simulink model "DIME12_Ctrl_dSpaceHRBMAB"  (R2018b)
settings: Solver=ode1  StartTime=0.0  StopTime=inf  FixedStep=0.5  RelTol=1e-3
PostLoadFcn:
  | if any(exist('dsrtsu_mdlpostloadfcn', 'file') ~= 0), dsrtsu_mdlpostloadfcn('Execute', bdroot); end
InitFcn:
  | , if any(exist('dsmpb_private', 'file') ~= 0), dsmpb_private('dsmpb_mdlclblib', 'Init', bdroot); end,
  | load('LUT_PSM.mat')
  | load('Torque_ts.mat')
  | 
  | p = 1;
  | L_q = 1.575e-3;
  | L_d = L_q;
  | Psi_M = 0.0353*2*pi;
  | R_s = 639e-3;
  | Ts = 1/40e3;
  | J_ges = 9.56e-5;
  | d_viskos = 0.01;
  | mpsTestMaxVelocityDmd = 166.7;
  | mpsTestVelocityDmd = 0;
  | EDC_CURRENT_CONTROL_EXECUTION_PERIOD = 4e-5;
  | 
undefined symbols (not defined in the file or in its folder): d, motor_KF, Psidq, Psiqd, q, SimSampleT
libraries: simulink x37, dsmpblib x12, simulink_extras x3
(part 2 of 2)

== system DIME12_Ctrl_dSpaceHRBMAB/DIME Regler/Controller/speed_controller/DISCRETE_PT1_SET ==
  Reset[0|1] : Inport
  In : Inport  Port=2
  K : Inport  Port=3
  T[s] : Inport  Port=4
  T_Sample[s] : Inport  Port=5
  1|FilterTime : Product  Inputs=*/  SaturateOnIntegerOverflow=on  InputSameDT=on  OutDataTypeStr=Inherit: Same as first input
  Proportional : Product  Inputs=**  SaturateOnIntegerOverflow=on  InputSameDT=on  OutDataTypeStr=Inherit: Same as first input
  Sum : Sum  Inputs=-+|  SaturateOnIntegerOverflow=on  InputSameDT=on  OutDataTypeStr=Inherit: Same as first input
  Unit Delay : UnitDelay  SampleTime=-1
  discrete_Integrator_Init : Subsystem
  zero : Constant  Value=0  SampleTime=-1
  Out : Outport
  wires:
  zero/1 -> discrete_Integrator_Init/3(Initial)
  T_Sample[s]/1 -> discrete_Integrator_Init/4(T_Sample[s])
  Reset[0|1]/1 -> discrete_Integrator_Init/1(Reset[0|1])
  T[s]/1 -> 1|FilterTime/2
  Unit Delay/1 -> Sum/1
  1|FilterTime/1 -> Unit Delay/1, Out/1
  discrete_Integrator_Init/1(Out) -> 1|FilterTime/1
  Proportional/1 -> Sum/2
  K/1 -> Proportional/2
  Sum/1 -> discrete_Integrator_Init/2(In)
  In/1 -> Proportional/1

== system DIME12_Ctrl_dSpaceHRBMAB/DIME Regler/Controller/speed_controller/DISCRETE_PT1_SET1 ==
  Reset[0|1] : Inport
  In : Inport  Port=2
  K : Inport  Port=3
  T[s] : Inport  Port=4
  T_Sample[s] : Inport  Port=5
  1|FilterTime : Product  Inputs=*/  SaturateOnIntegerOverflow=on  InputSameDT=on  OutDataTypeStr=Inherit: Same as first input
  Proportional : Product  Inputs=**  SaturateOnIntegerOverflow=on  InputSameDT=on  OutDataTypeStr=Inherit: Same as first input
  Sum : Sum  Inputs=-+|  SaturateOnIntegerOverflow=on  InputSameDT=on  OutDataTypeStr=Inherit: Same as first input
  Unit Delay : UnitDelay  SampleTime=-1
  discrete_Integrator_Init : Subsystem
  zero : Constant  Value=0  SampleTime=-1
  Out : Outport
  wires:
  zero/1 -> discrete_Integrator_Init/3(Initial)
  T_Sample[s]/1 -> discrete_Integrator_Init/4(T_Sample[s])
  Reset[0|1]/1 -> discrete_Integrator_Init/1(Reset[0|1])
  T[s]/1 -> 1|FilterTime/2
  Unit Delay/1 -> Sum/1
  1|FilterTime/1 -> Unit Delay/1, Out/1
  discrete_Integrator_Init/1(Out) -> 1|FilterTime/1
  Proportional/1 -> Sum/2
  K/1 -> Proportional/2
  Sum/1 -> discrete_Integrator_Init/2(In)
  In/1 -> Proportional/1

== system DIME12_Ctrl_dSpaceHRBMAB/DIME Regler/Controller/speed_controller/Limit_n_Set ==
  In1 : Inport
  In2 : Inport  Port=2
  Saturation Dynamic : simulink/Discontinuities/Saturation Dynamic  OutMin=[]  OutMax=[]  OutDataTypeStr=Inherit: Same as second input  OutDataType=sfix(16)  OutScaling=2^-10  DoSatur=off
  inv : Gain  Gain=-1
  Out1 : Outport
  wires:
  inv/1 -> Saturation Dynamic/3
  In2/1 -> Saturation Dynamic/1, inv/1
  In1/1 -> Saturation Dynamic/2
  Saturation Dynamic/1 -> Out1/1

== system DIME12_Ctrl_dSpaceHRBMAB/DIME Regler/Controller/speed_controller/PI_CONTROLLER ==
  ActualValue : Inport
  RefValue : Inport  Port=2
  Kp : Inport  Port=3
  Ki : Inport  Port=4
  Limit_up : Inport  Port=5
  Limit_lo : Inport  Port=6
  T_Sample[s] : Inport  Port=7
  Product : Product  RndMeth=Zero
  Product1 : Product  RndMeth=Zero
  Product2 : Product  RndMeth=Zero
  Saturation Dynamic : simulink/Discontinuities/Saturation Dynamic  OutMin=[]  OutMax=[]  OutDataTypeStr=Inherit: Same as second input  OutDataType=sfix(16)  OutScaling=2^-10  DoSatur=off
  Sum : Sum  Inputs=+++  SaturateOnIntegerOverflow=on
  Sum1 : Sum  Inputs=+-  SaturateOnIntegerOverflow=on
  Sum2 : Sum  Inputs=-+|  SaturateOnIntegerOverflow=on
  Unit Delay : UnitDelay  SampleTime=-1
  y : Outport
  wires:
  Limit_lo/1 -> Saturation Dynamic/3
  Limit_up/1 -> Saturation Dynamic/1
  Sum/1 -> Saturation Dynamic/2
  Sum1/1 -> Product1/2, Product2/1  "error"
  RefValue/1 -> Sum1/1
  ActualValue/1 -> Sum1/2
  Product1/1 -> Sum/1, Sum2/1
  Product/1 -> Sum/2  "integral"
  Saturation Dynamic/1 -> Sum2/2, y/1
  Product2/1 -> Product/1
  Unit Delay/1 -> Sum/3
  Sum2/1 -> Unit Delay/1
  T_Sample[s]/1 -> Product/2
  Kp/1 -> Product1/1
  Ki/1 -> Product2/2

== system DIME12_Ctrl_dSpaceHRBMAB/DIME Regler/Controller/speed_controller/SignalCollector ==
  n_Limit[rpm] : Inport
  n[rpm] : Inport  Port=2
  n_Set[rpm] : Inport  Port=3
  Bus Creator : BusCreator  Inputs=3
  SignalBus : Outport
  wires:
  n_Limit[rpm]/1 -> Bus Creator/3  "n_Limit[rpm]"
  Bus Creator/1 -> SignalBus/1  "SPEED_CONTROLLER"
  n_Set[rpm]/1 -> Bus Creator/2  "n_Set[rpm]"
  n[rpm]/1 -> Bus Creator/1  "n[rpm]"

== system DIME12_Ctrl_dSpaceHRBMAB/DIME Regler/Outputs/Error Protection/current U ==
  Iphase1 : Inport
  CurrentNegLimit : Constant  Value=-18
  CurrentPosLimit : Constant  Value=18
  Logical Operator1 : Logic  Operator=OR  AllPortsSameDT=off  OutDataTypeStr=boolean
  current max : RelationalOperator  Operator=>  OutDataTypeStr=boolean  RndMeth=Simplest
  current min : RelationalOperator  Operator=<  OutDataTypeStr=boolean  RndMeth=Simplest
  Inverter_Current_U_Fault : Outport
  wires:
  Logical Operator1/1 -> Inverter_Current_U_Fault/1  "Inverter_Current_U_Fault"
  current min/1 -> Logical Operator1/2
  CurrentPosLimit/1 -> current max/2
  CurrentNegLimit/1 -> current min/2
  current max/1 -> Logical Operator1/1
  Iphase1/1 -> current min/1, current max/1

== system DIME12_Ctrl_dSpaceHRBMAB/DIME Regler/Outputs/Error Protection/current V ==
  Iphase2 : Inport
  CurrentNegLimit : Constant  Value=-18
  CurrentPosLimit : Constant  Value=18
  Logical Operator1 : Logic  Operator=OR  AllPortsSameDT=off  OutDataTypeStr=boolean
  current max : RelationalOperator  Operator=>  OutDataTypeStr=boolean  RndMeth=Simplest
  current min : RelationalOperator  Operator=<  OutDataTypeStr=boolean  RndMeth=Simplest
  Inverter_Current_V_Fault : Outport
  wires:
  Logical Operator1/1 -> Inverter_Current_V_Fault/1  "Inverter_Current_V_Fault"
  current min/1 -> Logical Operator1/2
  CurrentPosLimit/1 -> current max/2
  CurrentNegLimit/1 -> current min/2
  current max/1 -> Logical Operator1/1
  Iphase2/1 -> current min/1, current max/1

== system DIME12_Ctrl_dSpaceHRBMAB/DIME Regler/Outputs/Error Protection/current W ==
  Iphase3 : Inport
  CurrentNegLimit : Constant  Value=-18
  CurrentPosLimit : Constant  Value=18
  Logical Operator1 : Logic  Operator=OR  AllPortsSameDT=off  OutDataTypeStr=boolean
  current max : RelationalOperator  Operator=>  OutDataTypeStr=boolean  RndMeth=Simplest
  current min : RelationalOperator  Operator=<  OutDataTypeStr=boolean  RndMeth=Simplest
  Inverter_Current_W_Fault : Outport
  wires:
  Iphase3/1 -> current max/1, current min/1
  current max/1 -> Logical Operator1/1
  CurrentNegLimit/1 -> current min/2
  CurrentPosLimit/1 -> current max/2
  current min/1 -> Logical Operator1/2
  Logical Operator1/1 -> Inverter_Current_W_Fault/1  "Inverter_Current_W_Fault"

== system DIME12_Ctrl_dSpaceHRBMAB/DIME Regler/Outputs/Error Protection/speed ==
  meclVelocityMAB : Inport
  Logical Operator : Logic  Operator=OR  AllPortsSameDT=off  OutDataTypeStr=boolean
  SpeedNegLimit : Constant  Value=-10000/60
  SpeedPosLimit : Constant  Value=10000/60  OutDataTypeStr=double
  rpm max : RelationalOperator  Operator=>  OutDataTypeStr=boolean  RndMeth=Simplest
  rpm min : RelationalOperator  Operator=<  OutDataTypeStr=boolean  RndMeth=Simplest
  Engine_Speed_Fault : Outport
  wires:
  SpeedNegLimit/1 -> rpm min/2
  SpeedPosLimit/1 -> rpm max/2
  meclVelocityMAB/1 -> rpm min/1, rpm max/1
  rpm max/1 -> Logical Operator/1
  rpm min/1 -> Logical Operator/2
  Logical Operator/1 -> Engine_Speed_Fault/1  "Engine_Speed_Fault"

== system DIME12_Ctrl_dSpaceHRBMAB/DIME Regler/Outputs/Error Protection/termperature ==
  Temperature : Inport
  Relational Operator : RelationalOperator  Operator=<  OutDataTypeStr=boolean  RndMeth=Simplest
  VTHlimit : Constant  Value=1.6
  Inverter_Temp_Fault : Outport
  wires:
  Temperature/1 -> Relational Operator/1
  VTHlimit/1 -> Relational Operator/2
  Relational Operator/1 -> Inverter_Temp_Fault/1  "Inverter_Temp_Fault"

== system DIME12_Ctrl_dSpaceHRBMAB/DIME Regler/Outputs/SVM/SPACE_VECTOR_MODULATOR ==
  v_Stator[a;b;c][V] : Inport
  Add : Sum  Inputs=+-
  Constant : Constant  Value=0.067
  DutyCycle : Scope
  Max : MinMax  Function=max  SaturateOnIntegerOverflow=on  InputSameDT=on
  Min : MinMax  SaturateOnIntegerOverflow=on  InputSameDT=on
  Saturation : Saturate  UpperLimit=1  LowerLimit=0
  Saturation1 : Saturate  UpperLimit=1  LowerLimit=0
  Sum : Sum  Inputs=+-|  SaturateOnIntegerOverflow=on
  Sum2 : Sum  Inputs=-++  SaturateOnIntegerOverflow=on
  Sum4 : Sum  Inputs=-+|  SaturateOnIntegerOverflow=on
  half : Gain  Gain=1/2  SaturateOnIntegerOverflow=on  OutDataTypeStr=Inherit: Same as input  ParamDataTypeStr=Inherit: Same as input
  one : Constant
  DutyCycle_HSD[a;b;c][0_1] : Outport
  wires:
  Min/1 -> Sum/2, Sum2/1
  Max/1 -> Sum/1
  Sum4/1 -> half/1
  Sum/1 -> Sum4/1
  one/1 -> Sum4/2
  Sum2/1 -> Saturation/1
  half/1 -> Sum2/3
  v_Stator[a;b;c][V]/1 -> Sum2/2, Max/1, Min/1
  Saturation/1 -> Add/1
  Constant/1 -> Add/2
  Add/1 -> Saturation1/1
  Saturation1/1 -> DutyCycle/1, DutyCycle_HSD[a;b;c][0_1]/1

== system DIME12_Ctrl_dSpaceHRBMAB/DIME Regler/Outputs/SVM/voltage transformation inverse clark ==
  alpha : Inport
  beta : Inport  Port=2
  Add2 : Sum
  Add3 : Sum  Inputs=+-
  Gain : Gain  Gain=200
  Gain1 : Gain  Gain=200
  Gain2 : Gain  Gain=200
  Mux : Mux  Inputs=3
  U_PhaseU : Scope
  U_PhaseV : Scope
  U_PhaseW : Scope
  minus half : Gain  Gain=-1/2
  one : Gain
  root 3 by 2 : Gain  Gain=sqrt(3)/2
  "[3]" : Outport
  wires:
  Add3/1 -> Gain2/1, Mux/3
  Add2/1 -> Gain1/1, Mux/2
  minus half/1 -> Add3/1, Add2/1
  root 3 by 2/1 -> Add3/2, Add2/2
  Mux/1 -> "[3]"/1  "[3]"
  beta/1 -> root 3 by 2/1
  alpha/1 -> one/1, minus half/1
  one/1 -> Gain/1, Mux/1
  Gain/1 -> U_PhaseU/1
  Gain1/1 -> U_PhaseV/1
  Gain2/1 -> U_PhaseW/1

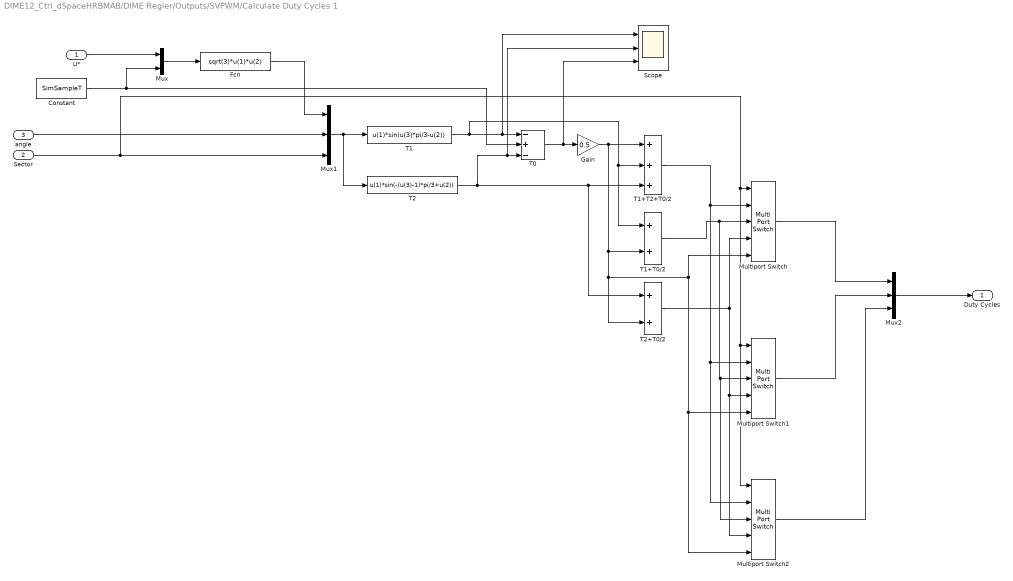
== system DIME12_Ctrl_dSpaceHRBMAB/DIME Regler/Outputs/SVPWM/Calculate Duty Cycles 1 ==
  U* : Inport
  Sector : Inport  Port=2
  angle : Inport  Port=3
  Constant : Constant  Value=SimSampleT
  Fcn : Fcn  Expr=sqrt(3)*u(1)*u(2)
  Gain : Gain  Gain=0.5
  Multiport Switch : MultiPortSwitch  DataPortOrder=Specify indices  Inputs=4  DataPortIndices={[1,6],2,5,[3,4]}
  Multiport Switch1 : MultiPortSwitch  DataPortOrder=Specify indices  Inputs=4  DataPortIndices={[2,3],4,1,[5,6]}
  Multiport Switch2 : MultiPortSwitch  DataPortOrder=Specify indices  Inputs=4  DataPortIndices={[4,5],6,3,[1,2]}
  Mux : Mux  Inputs=2
  Mux1 : Mux  Inputs=3
  Mux2 : Mux  Inputs=3
  Scope : Scope  NumInputPorts=3
  T0 : Sum  Inputs=-+-
  T1 : Fcn  Expr=u(1)*sin(u(3)*pi/3-u(2))
  T1+T0/2 : Sum
  T1+T2+T0/2 : Sum  Inputs=+++
  T2 : Fcn  Expr=u(1)*sin(-(u(3)-1)*pi/3+u(2))
  T2+T0/2 : Sum
  Duty Cycles : Outport
  wires:
  Mux/1 -> Fcn/1
  Constant/1 -> T0/2, Mux/2
  angle/1 -> Mux1/2
  Fcn/1 -> Mux1/1
  Sector/1 -> Multiport Switch2/1, Multiport Switch1/1, Multiport Switch/1, Mux1/3
  Mux1/1 -> T2/1, T1/1
  T1/1 -> T1+T0/2/1, T1+T2+T0/2/2, Scope/1, T0/1
  T2/1 -> T2+T0/2/1, T1+T2+T0/2/3, Scope/2, T0/3
  T0/1 -> Scope/3, Gain/1
  U*/1 -> Mux/1
  Gain/1 -> Multiport Switch2/5, Multiport Switch1/5, Multiport Switch/5, T2+T0/2/2, T1+T0/2/2, T1+T2+T0/2/1
  T1+T2+T0/2/1 -> Multiport Switch2/2, Multiport Switch1/2, Multiport Switch/2
  T1+T0/2/1 -> Multiport Switch2/3, Multiport Switch1/3, Multiport Switch/3
  T2+T0/2/1 -> Multiport Switch/4, Multiport Switch2/4, Multiport Switch1/4
  Multiport Switch/1 -> Mux2/1
  Multiport Switch1/1 -> Mux2/2
  Multiport Switch2/1 -> Mux2/3
  Mux2/1 -> Duty Cycles/1

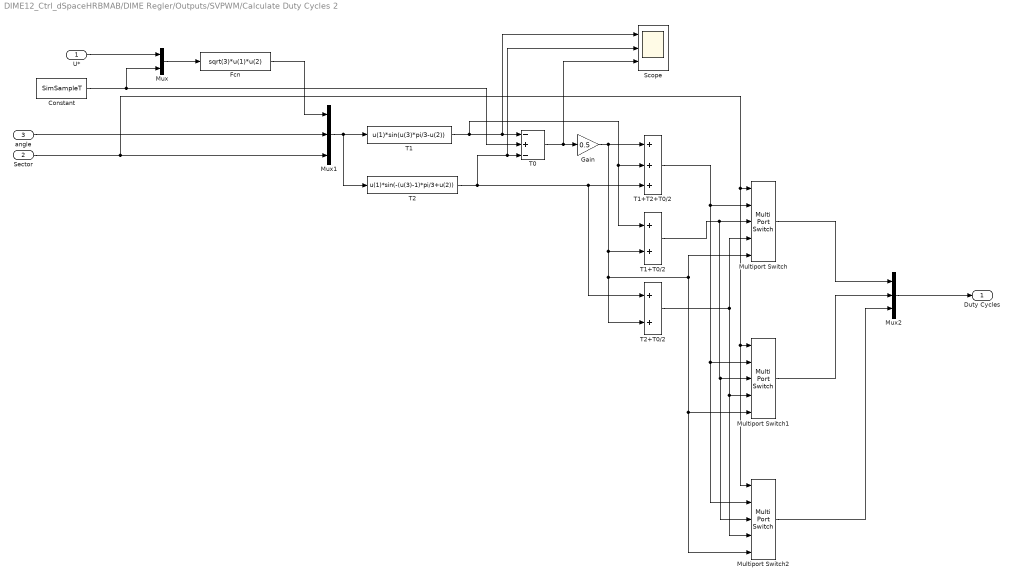
== system DIME12_Ctrl_dSpaceHRBMAB/DIME Regler/Outputs/SVPWM/Calculate Duty Cycles 2 ==
  U* : Inport
  Sector : Inport  Port=2
  angle : Inport  Port=3
  Constant : Constant  Value=SimSampleT
  Fcn : Fcn  Expr=sqrt(3)*u(1)*u(2)
  Gain : Gain  Gain=0.5
  Multiport Switch : MultiPortSwitch  DataPortOrder=Specify indices  Inputs=4  DataPortIndices={[1,6],2,5,[3,4]}
  Multiport Switch1 : MultiPortSwitch  DataPortOrder=Specify indices  Inputs=4  DataPortIndices={[2,3],4,1,[5,6]}
  Multiport Switch2 : MultiPortSwitch  DataPortOrder=Specify indices  Inputs=4  DataPortIndices={[4,5],6,3,[1,2]}
  Mux : Mux  Inputs=2
  Mux1 : Mux  Inputs=3
  Mux2 : Mux  Inputs=3
  Scope : Scope  NumInputPorts=3
  T0 : Sum  Inputs=-+-
  T1 : Fcn  Expr=u(1)*sin(u(3)*pi/3-u(2))
  T1+T0/2 : Sum
  T1+T2+T0/2 : Sum  Inputs=+++
  T2 : Fcn  Expr=u(1)*sin(-(u(3)-1)*pi/3+u(2))
  T2+T0/2 : Sum
  Duty Cycles : Outport
  wires:
  Mux2/1 -> Duty Cycles/1
  Multiport Switch2/1 -> Mux2/3
  Multiport Switch1/1 -> Mux2/2
  Multiport Switch/1 -> Mux2/1
  T2+T0/2/1 -> Multiport Switch1/4, Multiport Switch2/4, Multiport Switch/4
  T1+T0/2/1 -> Multiport Switch/3, Multiport Switch1/3, Multiport Switch2/3
  T1+T2+T0/2/1 -> Multiport Switch/2, Multiport Switch1/2, Multiport Switch2/2
  Gain/1 -> T1+T2+T0/2/1, T1+T0/2/2, T2+T0/2/2, Multiport Switch/5, Multiport Switch1/5, Multiport Switch2/5
  U*/1 -> Mux/1
  T0/1 -> Gain/1, Scope/3
  T2/1 -> T0/3, Scope/2, T1+T2+T0/2/3, T2+T0/2/1
  T1/1 -> T0/1, Scope/1, T1+T2+T0/2/2, T1+T0/2/1
  Mux1/1 -> T1/1, T2/1
  Sector/1 -> Mux1/3, Multiport Switch/1, Multiport Switch1/1, Multiport Switch2/1
  Fcn/1 -> Mux1/1
  angle/1 -> Mux1/2
  Constant/1 -> Mux/2, T0/2
  Mux/1 -> Fcn/1

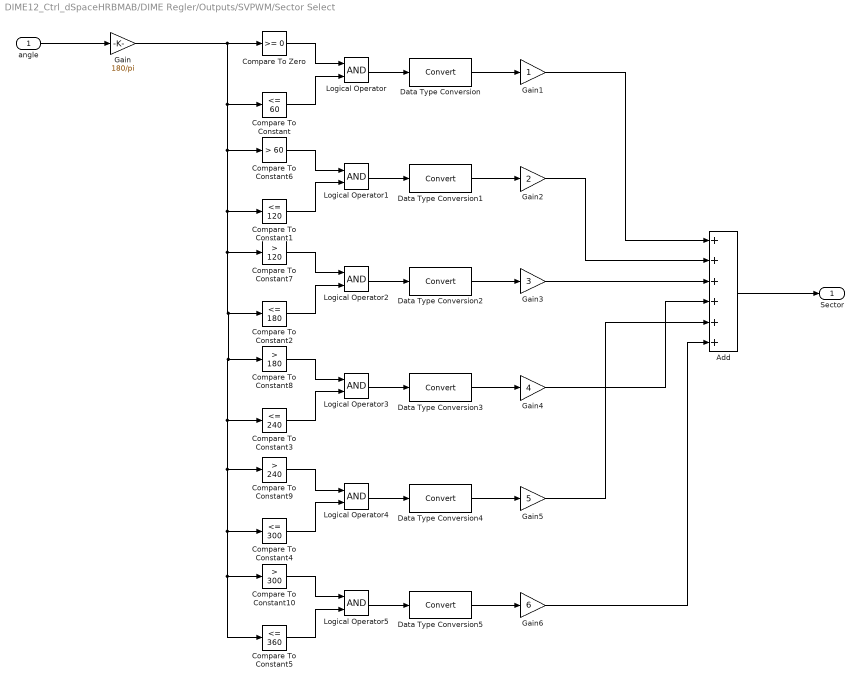
== system DIME12_Ctrl_dSpaceHRBMAB/DIME Regler/Outputs/SVPWM/Sector Select ==
  angle : Inport
  Add : Sum  Inputs=++++++
  Compare To Constant : simulink/Logic and Bit Operations/Compare To Constant  relop=<=  const=60  OutDataTypeStr=boolean
  Compare To Constant1 : simulink/Logic and Bit Operations/Compare To Constant  relop=<=  const=120  OutDataTypeStr=boolean
  Compare To Constant10 : simulink/Logic and Bit Operations/Compare To Constant  relop=>  const=300  OutDataTypeStr=boolean
  Compare To Constant2 : simulink/Logic and Bit Operations/Compare To Constant  relop=<=  const=180  OutDataTypeStr=boolean
  Compare To Constant3 : simulink/Logic and Bit Operations/Compare To Constant  relop=<=  const=240  OutDataTypeStr=boolean
  Compare To Constant4 : simulink/Logic and Bit Operations/Compare To Constant  relop=<=  const=300  OutDataTypeStr=boolean
  Compare To Constant5 : simulink/Logic and Bit Operations/Compare To Constant  relop=<=  const=360  OutDataTypeStr=boolean
  Compare To Constant6 : simulink/Logic and Bit Operations/Compare To Constant  relop=>  const=60  OutDataTypeStr=boolean
  Compare To Constant7 : simulink/Logic and Bit Operations/Compare To Constant  relop=>  const=120  OutDataTypeStr=boolean
  Compare To Constant8 : simulink/Logic and Bit Operations/Compare To Constant  relop=>  const=180  OutDataTypeStr=boolean
  Compare To Constant9 : simulink/Logic and Bit Operations/Compare To Constant  relop=>  const=240  OutDataTypeStr=boolean
  Compare To Zero : simulink/Logic and Bit Operations/Compare To Zero  relop=>=  OutDataTypeStr=boolean
  Data Type Conversion{,1..5} (6 alike) : DataTypeConversion
  Gain : Gain  Gain=180/pi
  Gain1 : Gain
  Gain2 : Gain  Gain=2
  Gain3 : Gain  Gain=3
  Gain4 : Gain  Gain=4
  Gain5 : Gain  Gain=5
  Gain6 : Gain  Gain=6
  Logical Operator{,1..5} (6 alike) : Logic  AllPortsSameDT=off  OutDataTypeStr=boolean
  Sector : Outport
  wires:
  angle/1 -> Gain/1
  Compare To Zero/1 -> Logical Operator/1
  Compare To Constant/1 -> Logical Operator/2
  Logical Operator/1 -> Data Type Conversion/1
  Data Type Conversion/1 -> Gain1/1
  Data Type Conversion1/1 -> Gain2/1
  Logical Operator1/1 -> Data Type Conversion1/1
  Compare To Constant1/1 -> Logical Operator1/2
  Compare To Constant6/1 -> Logical Operator1/1
  Compare To Constant7/1 -> Logical Operator2/1
  Compare To Constant2/1 -> Logical Operator2/2
  Logical Operator2/1 -> Data Type Conversion2/1
  Data Type Conversion2/1 -> Gain3/1
  Data Type Conversion3/1 -> Gain4/1
  Logical Operator3/1 -> Data Type Conversion3/1
  Compare To Constant3/1 -> Logical Operator3/2
  Compare To Constant8/1 -> Logical Operator3/1
  Compare To Constant9/1 -> Logical Operator4/1
  Compare To Constant4/1 -> Logical Operator4/2
  Logical Operator4/1 -> Data Type Conversion4/1
  Data Type Conversion4/1 -> Gain5/1
  Data Type Conversion5/1 -> Gain6/1
  Logical Operator5/1 -> Data Type Conversion5/1
  Compare To Constant5/1 -> Logical Operator5/2
  Compare To Constant10/1 -> Logical Operator5/1
  Gain/1 -> Compare To Constant6/1, Compare To Constant7/1, Compare To Constant9/1, Compare To Constant10/1, Compare To Constant5/1, Compare To Constant4/1, Compare To Constant3/1, Compare To Constant8/1, Compare To Constant2/1, Compare To Constant1/1, Compare To Constant/1, Compare To Zero/1
  Gain1/1 -> Add/1
  Gain2/1 -> Add/2
  Gain3/1 -> Add/3
  Gain4/1 -> Add/4
  Gain5/1 -> Add/5
  Gain6/1 -> Add/6
  Add/1 -> Sector/1

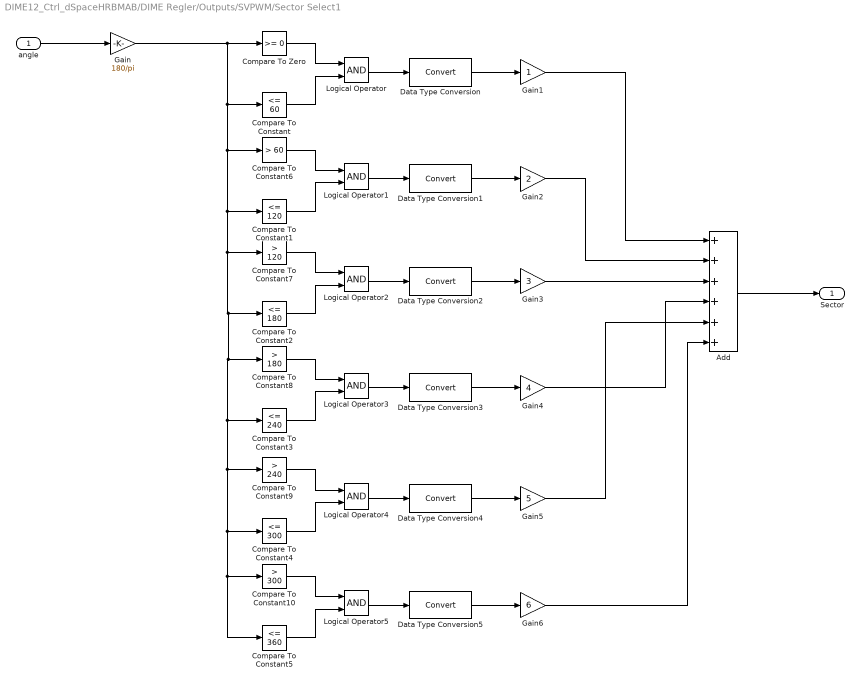
== system DIME12_Ctrl_dSpaceHRBMAB/DIME Regler/Outputs/SVPWM/Sector Select1 ==
  angle : Inport
  Add : Sum  Inputs=++++++
  Compare To Constant : simulink/Logic and Bit Operations/Compare To Constant  relop=<=  const=60  OutDataTypeStr=boolean
  Compare To Constant1 : simulink/Logic and Bit Operations/Compare To Constant  relop=<=  const=120  OutDataTypeStr=boolean
  Compare To Constant10 : simulink/Logic and Bit Operations/Compare To Constant  relop=>  const=300  OutDataTypeStr=boolean
  Compare To Constant2 : simulink/Logic and Bit Operations/Compare To Constant  relop=<=  const=180  OutDataTypeStr=boolean
  Compare To Constant3 : simulink/Logic and Bit Operations/Compare To Constant  relop=<=  const=240  OutDataTypeStr=boolean
  Compare To Constant4 : simulink/Logic and Bit Operations/Compare To Constant  relop=<=  const=300  OutDataTypeStr=boolean
  Compare To Constant5 : simulink/Logic and Bit Operations/Compare To Constant  relop=<=  const=360  OutDataTypeStr=boolean
  Compare To Constant6 : simulink/Logic and Bit Operations/Compare To Constant  relop=>  const=60  OutDataTypeStr=boolean
  Compare To Constant7 : simulink/Logic and Bit Operations/Compare To Constant  relop=>  const=120  OutDataTypeStr=boolean
  Compare To Constant8 : simulink/Logic and Bit Operations/Compare To Constant  relop=>  const=180  OutDataTypeStr=boolean
  Compare To Constant9 : simulink/Logic and Bit Operations/Compare To Constant  relop=>  const=240  OutDataTypeStr=boolean
  Compare To Zero : simulink/Logic and Bit Operations/Compare To Zero  relop=>=  OutDataTypeStr=boolean
  Data Type Conversion{,1..5} (6 alike) : DataTypeConversion
  Gain : Gain  Gain=180/pi
  Gain1 : Gain
  Gain2 : Gain  Gain=2
  Gain3 : Gain  Gain=3
  Gain4 : Gain  Gain=4
  Gain5 : Gain  Gain=5
  Gain6 : Gain  Gain=6
  Logical Operator{,1..5} (6 alike) : Logic  AllPortsSameDT=off  OutDataTypeStr=boolean
  Sector : Outport
  wires:
  Add/1 -> Sector/1
  Gain6/1 -> Add/6
  Gain5/1 -> Add/5
  Gain4/1 -> Add/4
  Gain3/1 -> Add/3
  Gain2/1 -> Add/2
  Gain1/1 -> Add/1
  Gain/1 -> Compare To Zero/1, Compare To Constant/1, Compare To Constant1/1, Compare To Constant2/1, Compare To Constant8/1, Compare To Constant3/1, Compare To Constant4/1, Compare To Constant5/1, Compare To Constant10/1, Compare To Constant9/1, Compare To Constant7/1, Compare To Constant6/1
  Compare To Constant10/1 -> Logical Operator5/1
  Compare To Constant5/1 -> Logical Operator5/2
  Logical Operator5/1 -> Data Type Conversion5/1
  Data Type Conversion5/1 -> Gain6/1
  Data Type Conversion4/1 -> Gain5/1
  Logical Operator4/1 -> Data Type Conversion4/1
  Compare To Constant4/1 -> Logical Operator4/2
  Compare To Constant9/1 -> Logical Operator4/1
  Compare To Constant8/1 -> Logical Operator3/1
  Compare To Constant3/1 -> Logical Operator3/2
  Logical Operator3/1 -> Data Type Conversion3/1
  Data Type Conversion3/1 -> Gain4/1
  Data Type Conversion2/1 -> Gain3/1
  Logical Operator2/1 -> Data Type Conversion2/1
  Compare To Constant2/1 -> Logical Operator2/2
  Compare To Constant7/1 -> Logical Operator2/1
  Compare To Constant6/1 -> Logical Operator1/1
  Compare To Constant1/1 -> Logical Operator1/2
  Logical Operator1/1 -> Data Type Conversion1/1
  Data Type Conversion1/1 -> Gain2/1
  Data Type Conversion/1 -> Gain1/1
  Logical Operator/1 -> Data Type Conversion/1
  Compare To Constant/1 -> Logical Operator/2
  Compare To Zero/1 -> Logical Operator/1
  angle/1 -> Gain/1

== system DIME12_Ctrl_dSpaceHRBMAB/DIME Regler/Outputs/SVPWM/reference U* ==
  note: Pha_U* (rad)
      | or
      | U* beta
  note: Mag_U*
      | or
      | U* alpha
  In1 : Inport
  In2 : Inport  Port=2
  "0<m<1 " : Saturate  UpperLimit=1  LowerLimit=0
  Cartesian to Polar : simulink_extras/Transformations/Cartesian to Polar
      settings: SourceProductName=Simulink
  Constant2 : Constant  Value=2*pi
  Math Function2 : Math  Operator=mod  SaturateOnIntegerOverflow=on
  Scope : Scope
  U* : Outport
  angle : Outport  Port=2
  wires:
  Cartesian to Polar/1 -> "0<m<1 "/1
  Cartesian to Polar/2 -> Math Function2/1
  Math Function2/1 -> Scope/1, angle/1
  Constant2/1 -> Math Function2/2
  "0<m<1 "/1 -> U*/1
  In1/1 -> Cartesian to Polar/1
  In2/1 -> Cartesian to Polar/2

== system DIME12_Ctrl_dSpaceHRBMAB/DIME Regler/Outputs/SVPWM/reference U*1 ==
  note: Mag_U*
      | or
      | U* alpha
  note: Pha_U* (rad)
      | or
      | U* beta
  In1 : Inport
  In2 : Inport  Port=2
  "0<m<1 " : Saturate  UpperLimit=1  LowerLimit=0
  Cartesian to Polar : simulink_extras/Transformations/Cartesian to Polar
      settings: SourceProductName=Simulink
  Constant2 : Constant  Value=2*pi
  Math Function2 : Math  Operator=mod  SaturateOnIntegerOverflow=on
  Scope : Scope
  U* : Outport
  angle : Outport  Port=2
  wires:
  In2/1 -> Cartesian to Polar/2
  In1/1 -> Cartesian to Polar/1
  "0<m<1 "/1 -> U*/1
  Constant2/1 -> Math Function2/2
  Math Function2/1 -> angle/1, Scope/1
  Cartesian to Polar/2 -> Math Function2/1
  Cartesian to Polar/1 -> "0<m<1 "/1

== system DIME12_Ctrl_dSpaceHRBMAB/DIME Regler/Controller/mpsTestMode/Velocitylimit/Subsystem ==
  unlimdInput : Inport
  Action Port : ActionPort  ActionType=else
  limdInput : Outport  InitialOutput=0
  wires:
  unlimdInput/1 -> limdInput/1

== system DIME12_Ctrl_dSpaceHRBMAB/DIME Regler/Controller/mpsTestMode/Velocitylimit/Subsystem1 ==
  LowerLimit : Inport
  Action Port : ActionPort  ActionType=elseif
  limdInput : Outport  InitialOutput=0
  wires:
  LowerLimit/1 -> limdInput/1

== system DIME12_Ctrl_dSpaceHRBMAB/DIME Regler/Controller/mpsTestMode/Velocitylimit/Subsystem2 ==
  UpperLimit : Inport
  Action Port : ActionPort  ActionType=then
  limdInput : Outport  InitialOutput=0
  wires:
  UpperLimit/1 -> limdInput/1

== system DIME12_Ctrl_dSpaceHRBMAB/DIME Regler/Controller/speed_controller/DISCRETE_PT1_SET/discrete_Integrator_Init ==
  Reset[0|1] : Inport
  In : Inport  Port=2
  Initial : Inport  Port=3
  T_Sample[s] : Inport  Port=4
  Add : Sum  Inputs=+++
  Compare To Constant : simulink/Logic and Bit Operations/Compare To Constant  relop===  const=0  OutDataTypeStr=uint8  ZeroCross=off
  Constant1 : Constant  Value=0
  Constant2 : Constant  Value=0
  Logical Operator : Logic  Operator=OR  AllPortsSameDT=off  OutDataTypeStr=boolean
  Product : Product  RndMeth=Zero
  Saturation : simulink/Discontinuities/Saturation Dynamic  OutMin=[]  OutMax=[]  OutDataTypeStr=Inherit: Same as second input  OutDataType=sfix(16)  OutScaling=2^-10  DoSatur=off
  Switch1 : Switch  Threshold=0.5
  Switch2 : Switch  Threshold=0.5
  Unit Delay : UnitDelay  SampleTime=-1
  Unit Delay1 : UnitDelay  SampleTime=-1
  lower_limit : Constant  Value=-1e300
  "only_rising_edge " : Subsystem
  upper_limit : Constant  Value=1e300
  Out : Outport
  wires:
  lower_limit/1 -> Saturation/3
  upper_limit/1 -> Saturation/1
  Saturation/1 -> Unit Delay/1, Out/1
  Add/1 -> Saturation/2
  T_Sample[s]/1 -> Product/1, Unit Delay1/1
  Product/1 -> Add/2
  Reset[0|1]/1 -> "only_rising_edge "/1(In1)
  In/1 -> Product/2
  Constant2/1 -> Switch2/1
  Switch2/1 -> Add/3
  Unit Delay/1 -> Switch2/3
  Switch1/1 -> Add/1
  Initial/1 -> Switch1/1
  Constant1/1 -> Switch1/3
  "only_rising_edge "/1(Out1) -> Logical Operator/2, Switch2/2
  Unit Delay1/1 -> Compare To Constant/1
  Logical Operator/1 -> Switch1/2
  Compare To Constant/1 -> Logical Operator/1

== system DIME12_Ctrl_dSpaceHRBMAB/DIME Regler/Controller/speed_controller/DISCRETE_PT1_SET1/discrete_Integrator_Init ==
  Reset[0|1] : Inport
  In : Inport  Port=2
  Initial : Inport  Port=3
  T_Sample[s] : Inport  Port=4
  Add : Sum  Inputs=+++
  Compare To Constant : simulink/Logic and Bit Operations/Compare To Constant  relop===  const=0  OutDataTypeStr=uint8  ZeroCross=off
  Constant1 : Constant  Value=0
  Constant2 : Constant  Value=0
  Logical Operator : Logic  Operator=OR  AllPortsSameDT=off  OutDataTypeStr=boolean
  Product : Product  RndMeth=Zero
  Saturation : simulink/Discontinuities/Saturation Dynamic  OutMin=[]  OutMax=[]  OutDataTypeStr=Inherit: Same as second input  OutDataType=sfix(16)  OutScaling=2^-10  DoSatur=off
  Switch1 : Switch  Threshold=0.5
  Switch2 : Switch  Threshold=0.5
  Unit Delay : UnitDelay  SampleTime=-1
  Unit Delay1 : UnitDelay  SampleTime=-1
  lower_limit : Constant  Value=-1e300
  "only_rising_edge " : Subsystem
  upper_limit : Constant  Value=1e300
  Out : Outport
  wires:
  lower_limit/1 -> Saturation/3
  upper_limit/1 -> Saturation/1
  Saturation/1 -> Unit Delay/1, Out/1
  Add/1 -> Saturation/2
  T_Sample[s]/1 -> Product/1, Unit Delay1/1
  Product/1 -> Add/2
  Reset[0|1]/1 -> "only_rising_edge "/1(In1)
  In/1 -> Product/2
  Constant2/1 -> Switch2/1
  Switch2/1 -> Add/3
  Unit Delay/1 -> Switch2/3
  Switch1/1 -> Add/1
  Initial/1 -> Switch1/1
  Constant1/1 -> Switch1/3
  "only_rising_edge "/1(Out1) -> Logical Operator/2, Switch2/2
  Unit Delay1/1 -> Compare To Constant/1
  Logical Operator/1 -> Switch1/2
  Compare To Constant/1 -> Logical Operator/1

== system DIME12_Ctrl_dSpaceHRBMAB/DIME Regler/Controller/speed_controller/DISCRETE_PT1_SET/discrete_Integrator_Init/only_rising_edge  ==
  In1 : Inport
  Compare To Constant1 : simulink/Logic and Bit Operations/Compare To Constant  relop===  const=0  OutDataTypeStr=uint8  ZeroCross=off
  Compare To Constant2 : simulink/Logic and Bit Operations/Compare To Constant  relop===  const=1  OutDataTypeStr=uint8  ZeroCross=off
  Logical Operator1 : Logic  AllPortsSameDT=off  OutDataTypeStr=boolean
  Unit Delay2 : UnitDelay  SampleTime=-1
  Out1 : Outport
  wires:
  Unit Delay2/1 -> Compare To Constant1/1
  In1/1 -> Unit Delay2/1, Compare To Constant2/1
  Compare To Constant1/1 -> Logical Operator1/1
  Compare To Constant2/1 -> Logical Operator1/2
  Logical Operator1/1 -> Out1/1

== system DIME12_Ctrl_dSpaceHRBMAB/DIME Regler/Controller/speed_controller/DISCRETE_PT1_SET1/discrete_Integrator_Init/only_rising_edge  ==
  In1 : Inport
  Compare To Constant1 : simulink/Logic and Bit Operations/Compare To Constant  relop===  const=0  OutDataTypeStr=uint8  ZeroCross=off
  Compare To Constant2 : simulink/Logic and Bit Operations/Compare To Constant  relop===  const=1  OutDataTypeStr=uint8  ZeroCross=off
  Logical Operator1 : Logic  AllPortsSameDT=off  OutDataTypeStr=boolean
  Unit Delay2 : UnitDelay  SampleTime=-1
  Out1 : Outport
  wires:
  Unit Delay2/1 -> Compare To Constant1/1
  In1/1 -> Unit Delay2/1, Compare To Constant2/1
  Compare To Constant1/1 -> Logical Operator1/1
  Compare To Constant2/1 -> Logical Operator1/2
  Logical Operator1/1 -> Out1/1

== matlab function DIME12_Ctrl_dSpaceHRBMAB/DIME Regler/Controller/ParkClarke ==
  data: vd input; vq input; theta input; valpha output; vbeta output
function [valpha,vbeta] = fcn(vd,vq,theta)

%iabc = (2/3)*[1, 0; -0.5, sqrt(3)/2; -0.5, -sqrt(3)/2]*([cos(theta), -sin(theta); sin(theta), cos(theta)]*[id; iq]);
valpha=vd*cos(theta) -vq*sin(theta);
vbeta =vd*sin(theta) +vq*cos(theta);

% ia = iabc(1);
% ib = iabc(2);
% ic = iabc(3);

== matlab function DIME12_Ctrl_dSpaceHRBMAB/DIME Regler/Controller/Decoupling ==
  data: iq input; yd output; p input; w input; Lq input; id input; Ld input; yq output; phi input
function [yd,yq] = fcn(iq,p,w,Lq,id,Ld,phi)

yd= -iq*w*p*Lq;

yq= id*w*p*Ld +phi*p*w;

== matlab function DIME12_Ctrl_dSpaceHRBMAB/DIME Regler/Controller/MATLAB Function ==
  data: T input; iq output
function iq = fcn(T)
p=1;
Psi_M = 0.0353*2*pi;
iq = T/(3/2* p *Psi_M);

== matlab function DIME12_Ctrl_dSpaceHRBMAB/DIME Regler/Controller/Identifier_AnyTask/NN Identifier ==
  settings: updateMethod=DISCRETE
  data: h input; id input; iq input; ud input; uq input; omega input; R output; d_id input; d_iq input; Gamma_Theta_R input; Gamma_W_R input; psi_m0 output; J output; Gamma_Theta_psi input; Gamma_W_psi input; takeover input; psim0_est input
function [R, psi_m0, J] = Approximate(h,id,iq,ud,uq,omega, d_id, d_iq, ...
    Gamma_Theta_R, Gamma_W_R,  Gamma_Theta_psi, Gamma_W_psi, takeover, psim0_est )

    % % HRB nominal parameters 
    % Psi_M = 0.0353*2*pi;
    % R_s = 639e-3;


 
if(1)
    Gamma_Theta_ldq10=0;
    Gamma_W_ldq10 = 0;
end
if(1)
    Gamma_Theta_lqd10=0;
    Gamma_W_lqd10 = 0;
end
 




persistent W_R_T ...
           W_l_qd10_T ...
           W_l_dq10_T ...
           W_psi_m0_T ...
           Theta_R_T ...
           Theta_l_qd10_T ...
           Theta_l_dq10_T ...
           Theta_psi_m0_T ...


if isempty(W_R_T) || isempty(W_l_qd10_T) || isempty(W_l_dq10_T) ||  isempty(W_psi_m0_T) || isempty(Theta_R_T) || isempty(Theta_l_qd10_T)  || isempty(Theta_l_dq10_T) ||  isempty(Theta_psi_m0_T)      
 
 
W_R_T = [2.04822644461840e-05,2.04816119048058e-05;2.04823577258696e-05,2.04822462184732e-05;2.04815774888327e-05,2.04817617170584e-05;2.04823629611794e-05,2.04819781184588e-05;2.04820849325778e-05,2.04816182220611e-05;2.04815497917300e-05,2.04820542332664e-05;2.04817290895107e-05,2.04817135625764e-05;2.04819978477042e-05,2.04821050452835e-05;2.04824082972273e-05,2.04821400048950e-05;2.04824137487725e-05,2.04821970118301e-05];
 
Theta_R_T = [0.0179437411497698	0.00897193402779521	0.00897193446402229	0.00897193417960009	0.00897193400199923	0.00897193458740008	0.00897193452389927	0.00897193419739507	0.00897193427267327	0.00897193423924112	0.00897193386022727];
 
W_psi_m0_T = [3.36596323929511e-07,3.35943782551311e-07;3.36687643195459e-07,3.36576135799067e-07;3.35908676332707e-07,3.36092904558458e-07;3.36694960020311e-07,3.36310117299679e-07;3.36414284189910e-07,3.35947573673185e-07;3.35879428791493e-07,3.36383870327895e-07;3.36060197795233e-07,3.36044670860906e-07;3.36328623112877e-07,3.36435820692149e-07;3.36739227973001e-07,3.36470935640707e-07;3.36746389889419e-07,3.36529652947043e-07];
 
Theta_psi_m0_T  = [0.00231788201112145	0.00115894119229074	0.00115894162568093	0.00115894134619483	0.00115894116467780	0.00115894175257942	0.00115894168946356	0.00115894136358532	0.00115894143628631	0.00115894140111420	0.00115894102185007];
 
Theta_l_dq10_T = [3.06272108646170e-05	1.53136618898215e-05	1.53140948664430e-05	1.53138161019030e-05	1.53136340111074e-05	1.53142222806330e-05	1.53141592211266e-05	1.53138334334557e-05	1.53139057572415e-05	1.53138703302795e-05	1.53134910283740e-05];
 
Theta_l_qd10_T = [3.61010730022179e-05	2.24659001336882e-05	2.24663328343095e-05	2.24660542446031e-05	2.24658722745621e-05	2.24664601632891e-05	2.24663971440134e-05	2.24660715653744e-05	2.24661438450041e-05	2.24661084424157e-05	2.24657293848019e-05];
 
W_l_dq10_T = [8.14669546231156e-10,1.62128168031204e-10;9.05741112018515e-10,7.94233715626875e-10;1.26933856909712e-10,3.11162082660982e-10;9.13321502492780e-10,5.28478781859986e-10;6.32309396785878e-10,1.65598880060266e-10;9.74900727413724e-11,6.01931609143709e-10;2.78445392179253e-10,2.62918457852358e-10;5.46829246235578e-10,6.54026825507379e-10;9.57454291187415e-10,6.89161958893324e-10;9.64833086769558e-10,7.48096144394093e-10];
 
W_l_qd10_T = [-0.000643412476326285,-0.000643413128867663;-0.000643412385485832,-0.000643412496993229;-0.000643413163888063,-0.000643412979659837;-0.000643412377824077,-0.000643412762666797;-0.000643412658626792,-0.000643413125337309;-0.000643413193414641,-0.000643412688973105;-0.000643413012409694,-0.000643413027936628;-0.000643412744237816,-0.000643412637040237;-0.000643412333756349,-0.000643412602048681;-0.000643412326400265,-0.000643412543137207];


end

 
x=1;    
 

x_bar = [1,x]';


 
L_q = 1.575e-3;
L_d = L_q;



R      = Theta_R_T      * Phi_1_T( W_R_T * x_bar )  ;

l_qd10 = L_q ;

l_dq10 = L_d ;

psi_m0 = Theta_psi_m0_T * Phi_1_T( W_psi_m0_T * x_bar ) ;

if(takeover)
psi_m0=psim0_est;
end

l_dq20 = 0; 
l_dq30 = 0; 
l_qd30 = 0; 
c_dq01 = 0;  
c_dq11 = 0;  

 
 
ud_hat = R*id - omega * ( l_qd10*iq + l_qd30*iq^3 + c_dq01*id*iq + 0.5*c_dq11*id^2*iq ) + (l_dq10 + 2*l_dq20*id + 3*l_dq30*id^2 + 0.5*c_dq11*iq^2) *  d_id;

uq_hat = R*iq + omega * ( psi_m0 + 0.5*c_dq01*iq^2 + l_dq10*id + l_dq20*id^2 + l_dq30*id^3 + 0.5*c_dq11*id*iq^2 ) + ( l_qd10 + 3*l_qd30*iq^2 + c_dq01*id + 0.5*c_dq11*id^2 ) * d_iq;

J = 0.5 * (ud_hat - ud)^2 + 0.5 * (uq_hat - uq)^2 ;

DJd = ud_hat - ud;
DJq = uq_hat - uq;

 


J_Theta_R_T      = Phi_1_T( W_R_T      * x_bar ) * (DJd * id                                   + DJq * iq);
J_Theta_l_qd10_T = Phi_1_T( W_l_qd10_T * x_bar ) * (DJd * (-omega*iq)                          + DJq * d_iq);
J_Theta_l_dq10_T = Phi_1_T( W_l_dq10_T * x_bar ) * (DJd * ( d_id )                             + DJq * ( id )* omega ) ;
J_Theta_psi_m0_T = Phi_1_T( W_psi_m0_T * x_bar ) * (                                             DJq * ( omega ));

  
J_W_R_T      = x_bar *( Theta_R_T(2:end)      * diag( dsigma( W_R_T      * x_bar ) ) * ( DJd * ( id )                                 + DJq * ( iq ) ) ); % 8x1 * 1x3 = 8x3
J_W_l_qd10_T = x_bar *( Theta_l_qd10_T(2:end) * diag( dsigma( W_l_qd10_T * x_bar ) ) * ( DJd * ( -omega*iq )                          + DJq * ( d_iq ) ) ); 
J_W_l_dq10_T = x_bar *( Theta_l_dq10_T(2:end) * diag( dsigma( W_l_dq10_T * x_bar ) ) * ( DJd * ( d_id )                               + DJq * ( omega*id ) ) ); 
J_W_psi_m0_T = x_bar *( Theta_psi_m0_T(2:end) * diag( dsigma( W_psi_m0_T * x_bar ) ) * (                                                DJq * ( omega ) ) ); 


Theta_R_T      = Theta_R_T      - 5e2*Gamma_Theta_R * J_Theta_R_T'      * h; 
Theta_l_qd10_T = Theta_l_qd10_T -  .2*Gamma_Theta_lqd10 * J_Theta_l_qd10_T'    * h; 
Theta_l_dq10_T = Theta_l_dq10_T -  .00005*Gamma_Theta_ldq10 * J_Theta_l_dq10_T' * h; 
Theta_psi_m0_T = Theta_psi_m0_T - 1*Gamma_Theta_psi * J_Theta_psi_m0_T'   * h;  

 
W_R_T      = W_R_T      - 5e2*Gamma_W_lqd10 * J_W_R_T'      * h; 
W_l_qd10_T = W_l_qd10_T - .2*Gamma_W_R * J_W_l_qd10_T' * h; 
W_l_dq10_T = W_l_dq10_T - .00005*Gamma_W_ldq10 * J_W_l_dq10_T' * h; 
W_psi_m0_T = W_psi_m0_T - 1*Gamma_W_psi * J_W_psi_m0_T' * h; 

  
 


 

function ds = dsigma(x)
a = 1;
ds = a*exp(-a*x)./( 1 + exp(-a*x) ).^2;
end

function Sigma = Phi_1_T(x)
a = 1;
s = 1./( 1 + exp(-a*x) );
Sigma = [1;s];
end

 

 


end

== matlab function DIME12_Ctrl_dSpaceHRBMAB/DIME Regler/dSpace Measurement/Inc Position Input/Moving Average ==
  data: y input; ymean output
function ymean = fcn( y )
persistent buf n buffull ;
ws = 500 ; % moving average window

% if isempty(buf)
% winSum = zeros(numel(y), 1) ;
% buf = zeros(numel(y), ws) ;
% n = 1 ;
% end
%
% winSum = winSum - buf(:, n) ; % delete oldest value
% winSum = winSum + y ; % add new value
% ymean = winSum ./ min(n, ws) ; % if n ws
% n = 1;
% end

if isempty(n)
n = 1 ;
buf = zeros(numel(y), ws) ;
buffull = 0 ;
end

buf(:, n) = y ;

ymean = y ;
if buffull % averaging only starts after buffer full
ymean = mean(buf, 2) ;
end

n = n + 1;
if n > ws
n = 1 ;
buffull = 1 ;
end

end

== matlab function DIME12_Ctrl_dSpaceHRBMAB/DIME Regler/Controller/ClarkePark ==
  data: ia input; id output; ib input; ic input; theta input; iq output; ids output; iqs output
function [ id,iq, ids, iqs] = fcn(ia,ib,ic,theta)

ids = (2/3)*( ia - ib/2 -ic/2 );
iqs = (2/3)*(sqrt(3)/2 * ib -  sqrt(3)/2*ic );

 
id = cos(theta)*ids + sin(theta)*iqs;
iq = -sin(theta)*ids + cos(theta)*iqs;
